simulink model "QuarterCar_LQR_Control"  (R2023b)
settings: Solver=VariableStepAuto  StartTime=0.0  StopTime=5  RelTol=1e-3
values from neighbouring files (symbols this model uses):
  A = [0 1 0 0 ... (first row only)    [LQR.m]
  B = [0 0 ... (first row only)    [LQR.m]
  C = [1 0 0 0 ... (first row only)    [LQR.m]
  D = [0 0 ... (first row only)    [LQR.m]
  K = K_LQR    [LQR.m]
  X0 = zeros(4,1)    [LQR.m]
  zr = 5e-2    (= 0.05)    [LQR.m]
settings Model: Creator=FawaD KhaN  LastModifiedBy=Muazu Modibbo
settings OptimizationCC: ReuseModelBlockBuffer=off

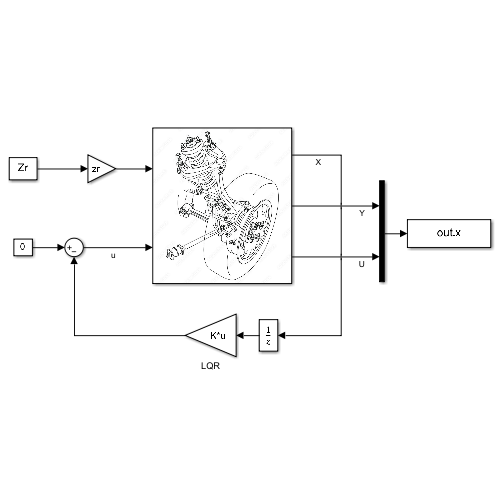
[thumbnail: Simulink's stored preview of the top-level diagram]
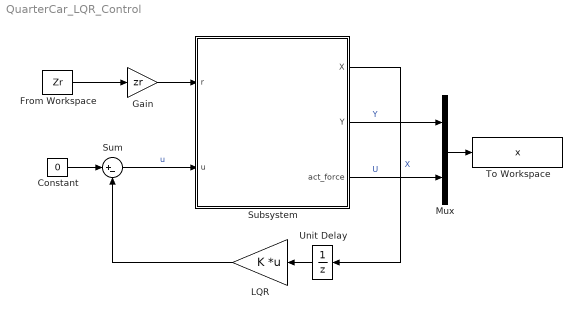
== system QuarterCar_LQR_Control ==
  Constant : Constant  Value=0
  From Workspace : FromWorkspace  VariableName=Zr
  Gain : Gain  Gain=zr
  LQR : Gain  Gain=K  Multiplication=Matrix(K*u)
  Mux : Mux  Inputs=2
  Subsystem : Subsystem
      mask Display: image('1000_F_372837830_pm8UAhDRhs7mo4GGVEQFyKpNt1jq0Z0f.jpg');
  Sum : Sum  Inputs=|+-
  To Workspace : ToWorkspace  VariableName=x  SampleTime=-1
      settings: Save2DSignal=2-D array (concatenate along first dimension)
  Unit Delay : UnitDelay  SampleTime=-1  HasFrameUpgradeWarning=on
  wires:
  Sum/1 -> Subsystem/2(u)  "u"
  Subsystem/1(X) -> Unit Delay/1  "X"
  Subsystem/3(act_force) -> Mux/2  "U"
  Subsystem/2(Y) -> Mux/1  "Y"
  Mux/1 -> To Workspace/1
  Constant/1 -> Sum/1
  From Workspace/1 -> Gain/1
  Unit Delay/1 -> LQR/1
  Gain/1 -> Subsystem/1(r)
  LQR/1 -> Sum/2

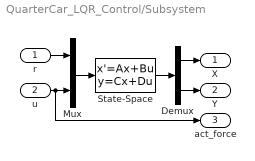
== system QuarterCar_LQR_Control/Subsystem ==
  r : Inport
  u : Inport  Port=2
  Demux : Demux  Outputs=[4,3]
  Mux : Mux  Inputs=2
  State-Space : StateSpace  A=A  B=B  C=[eye(4);C]  D=[zeros(4,2);D]  InitialCondition=X0  ParameterTunability=Unconstrained
  X : Outport
  Y : Outport  Port=2
  act_force : Outport  Port=3
  wires:
  r/1 -> Mux/1
  Mux/1 -> State-Space/1
  Demux/2 -> Y/1
  u/1 -> act_force/1, Mux/2
  State-Space/1 -> Demux/1
  Demux/1 -> X/1
